simulink model "PIDController"  (R2016b)
settings: Solver=VariableStepAuto  StartTime=0.0  StopTime=10.0  RelTol=1e-3
undefined symbols (not defined in the file): Kd, Ki, Kp
settings Model: Creator=1026691  LastModifiedBy=1026691

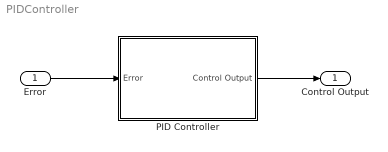
== system PIDController ==
  Error : Inport
  PID Controller : Subsystem
  Control Output : Outport
  wires:
  Error/1 -> PID Controller/1(Error)
  PID Controller/1(Control Output) -> Control Output/1

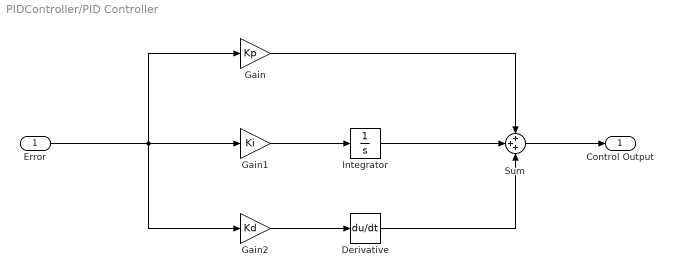
== system PIDController/PID Controller ==
  Error : Inport
  Derivative : Derivative
  Gain : Gain  Gain=Kp
  Gain1 : Gain  Gain=Ki
  Gain2 : Gain  Gain=Kd
  Integrator : Integrator
  Sum : Sum  Inputs=+++
  Control Output : Outport
  wires:
  Gain/1 -> Sum/1
  Gain1/1 -> Integrator/1
  Integrator/1 -> Sum/2
  Sum/1 -> Control Output/1
  Gain2/1 -> Derivative/1
  Derivative/1 -> Sum/3
  Error/1 -> Gain2/1, Gain1/1, Gain/1
